simulink library "send"  (R2024a)
settings: Solver=VariableStepAuto  StartTime=0.0  StopTime=10.0  RelTol=1e-3
settings Model: Creator=eikel  LastModifiedBy=eikel

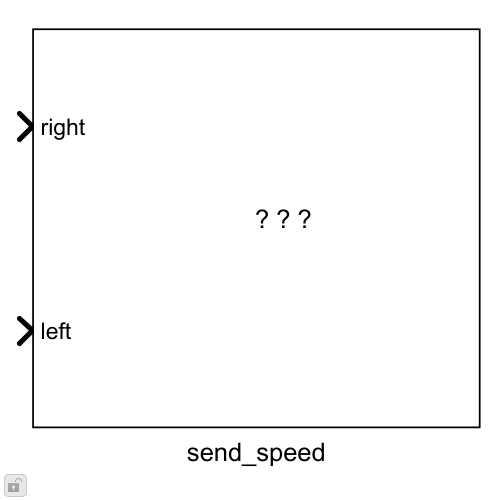
[thumbnail: Simulink's stored preview of the top-level diagram]
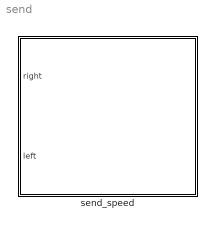
== system send ==
  send_speed : Subsystem
      mask Display: image('speed.jpg');

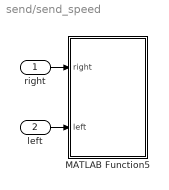
== system send/send_speed ==
  right : Inport
  left : Inport  Port=2
  MATLAB Function5 : MATLAB Function  TreatAsAtomicUnit=on
  wires:
  left/1 -> MATLAB Function5/2(left)
  right/1 -> MATLAB Function5/1(right)

== matlab function send/send_speed/MATLAB Function5 ==
  data: right input; left input
function publish_speed(right, left)
    coder.extrinsic('send_speed');  % merk: dette peikar på .m-fila di
    send_speed(right, left)
end
